simulink model "flight_dynamics_4"  (R2016b)
settings: Solver=FixedStepAuto  StartTime=0.0  StopTime=inf  FixedStep=.0005  RelTol=1e-3  EnableMultiTasking=on
InitFcn:
  | param
undefined symbols (not defined in the file): drawAircraft, forces_moments, P
libraries: simulink x4
settings Model: Creator=nmd89  LastModifiedBy=nmd89
settings OptimizationCC: LifeSpan=inf
settings DebuggingCC: SFUnexpectedBacktrackingDiag=warning  SFNoUnconditionalDefaultTransitionDiag=warning  SFExecutionAtInitializationDiag=none
settings GRTTargetCC: TargetLangStandard=C89/C90 (ANSI)  GeneratePreprocessorConditionals=Disable all
settings ConfigComp: CovMetricSettings=dw  CovHtmlReporting=on  CovSaveCumulativeToWorkspaceVar=on  CovSaveSingleToWorkspaceVar=on  CovExternalEMLEnable=off

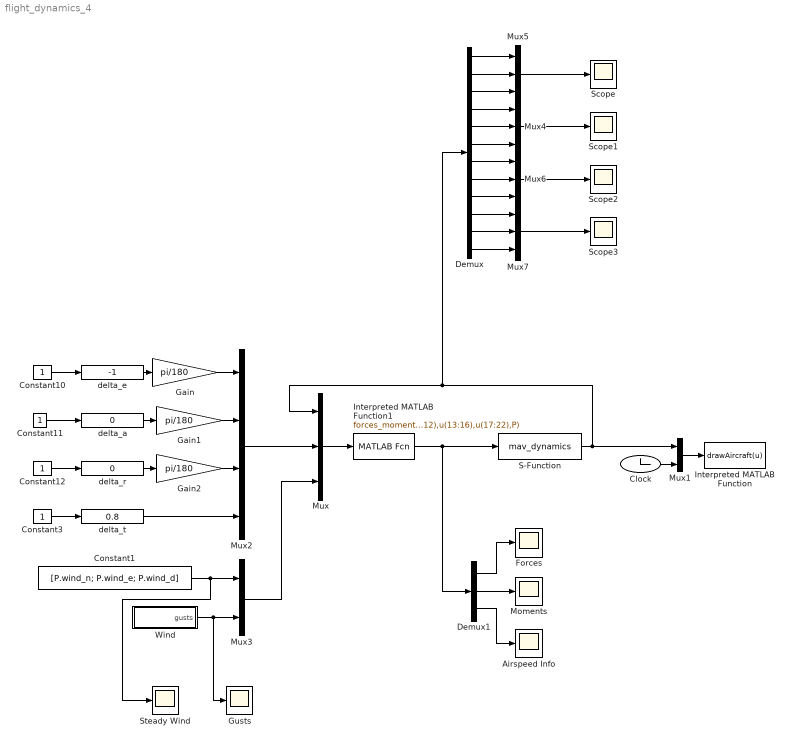
== system flight_dynamics_4 ==
  Airspeed Info : Scope
  Clock : Clock
  Constant1 : Constant  Value=[P.wind_n; P.wind_e; P.wind_d]
  Constant{3,10..12} (4 alike) : Constant
  Demux : Demux  Outputs=12
  Demux1 : Demux  Outputs=[3;3;6]
  Forces : Scope
  Gain : Gain  Gain=pi/180
  Gain1 : Gain  Gain=pi/180
  Gain2 : Gain  Gain=pi/180
  Gusts : Scope
  Interpreted MATLAB Function : MATLABFcn  MATLABFcn=drawAircraft(u)  OutputDimensions=0
  Interpreted MATLAB Function1 : MATLABFcn  MATLABFcn=forces_moments(u(1:12),u(13:16),u(17:22),P)
  Moments : Scope
  Mux{,4..7} (5 alike) : Mux  Inputs=3
  Mux1 : Mux  Inputs=2
  Mux2 : Mux
  Mux3 : Mux  Inputs=2
  S-Function : S-Function  FunctionName=mav_dynamics  Parameters=P  SFunctionDeploymentMode=off  EnableBusSupport=off
  Scope{,1..3} (4 alike) : Scope
  Steady Wind : Scope
  Wind : Subsystem
  delta_a : simulink/Math Operations/Slider Gain  low=-45  gain=0  high=45
  delta_e : simulink/Math Operations/Slider Gain  low=-45  gain=-1  high=45
  delta_r : simulink/Math Operations/Slider Gain  low=-45  gain=0  high=45
  delta_t : simulink/Math Operations/Slider Gain  low=0  gain=0.8  high=1
  wires:
  Mux1/1 -> Interpreted MATLAB Function/1
  Clock/1 -> Mux1/2
  S-Function/1 -> Demux/1, Mux/1, Mux1/1
  Mux/1 -> Interpreted MATLAB Function1/1
  Mux2/1 -> Mux/2
  Mux3/1 -> Mux/3
  Wind/1(gusts) -> Gusts/1, Mux3/2
  Constant1/1 -> Steady Wind/1, Mux3/1
  Constant10/1 -> delta_e/1
  Constant11/1 -> delta_a/1
  Constant12/1 -> delta_r/1
  delta_r/1 -> Gain2/1
  delta_a/1 -> Gain1/1
  delta_e/1 -> Gain/1
  Constant3/1 -> delta_t/1
  delta_t/1 -> Mux2/4
  Gain1/1 -> Mux2/2
  Gain2/1 -> Mux2/3
  Gain/1 -> Mux2/1
  Interpreted MATLAB Function1/1 -> Demux1/1, S-Function/1
  Demux/4 -> Mux4/1
  Demux/5 -> Mux4/2
  Demux/6 -> Mux4/3
  Mux4/1 -> Scope1/1
  Demux/1 -> Mux5/1
  Demux/2 -> Mux5/2
  Demux/3 -> Mux5/3
  Mux5/1 -> Scope/1
  Mux6/1 -> Scope2/1
  Demux/7 -> Mux6/1
  Demux/8 -> Mux6/2
  Demux/9 -> Mux6/3
  Mux7/1 -> Scope3/1
  Demux/10 -> Mux7/1
  Demux/11 -> Mux7/2
  Demux/12 -> Mux7/3
  Demux1/1 -> Forces/1
  Demux1/2 -> Moments/1
  Demux1/3 -> Airspeed Info/1

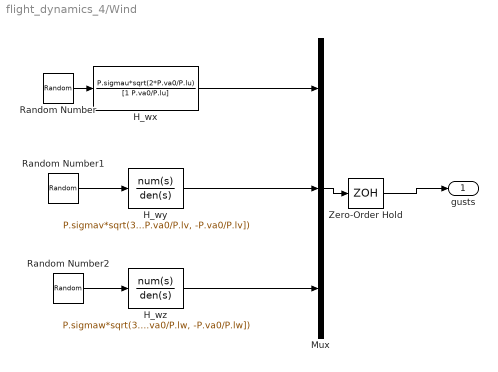
== system flight_dynamics_4/Wind ==
  H_wx : TransferFcn  Numerator=P.sigmau*sqrt(2*P.va0/P.lu)  Denominator=[1 P.va0/P.lu]
  H_wy : TransferFcn  Numerator=P.sigmav*sqrt(3*P.va0/P.lv)*[0, 1, P.va0/sqrt(3)/P.lv]  Denominator=poly([-P.va0/P.lv, -P.va0/P.lv])
  H_wz : TransferFcn  Numerator=P.sigmaw*sqrt(3*P.va0/P.lw)*[0, 1, P.va0/sqrt(3)/P.lw]  Denominator=poly([-P.va0/P.lw, -P.va0/P.lw])
  Mux : Mux  Inputs=3
  Random Number : RandomNumber  SampleTime=0
  Random Number1 : RandomNumber  SampleTime=0
  Random Number2 : RandomNumber  SampleTime=0
  Zero-Order Hold : ZeroOrderHold  SampleTime=P.Ts
  gusts : Outport
  wires:
  H_wx/1 -> Mux/1
  Random Number/1 -> H_wx/1
  H_wy/1 -> Mux/2
  Random Number1/1 -> H_wy/1
  H_wz/1 -> Mux/3
  Random Number2/1 -> H_wz/1
  Mux/1 -> Zero-Order Hold/1
  Zero-Order Hold/1 -> gusts/1
